simulink model "p5p5ex"  (Simulink 9.2)
settings: Solver=ode45  StartTime=0.0  StopTime=1000  RelTol=1e-3  EnableMultiTasking=on
values from neighbouring files (symbols this model uses):
  Kpd = 0.8427    [p5p5c.m]    (also in p5p5d.m; p5p5e.m)
  Td = T    (= 72.4391)    [p5p5c.m]    (also in p5p5d.m; p5p5e.m)
  Tf = 8.391    [p5p5c.m]    (also in p5p5d.m; p5p5e.m)
libraries: simulink x2
settings Model: Creator=markh  LastModifiedBy=Kevin K. Kaldvansvik
settings DataIOCC: SignalLoggingName=sigsOut
settings OptimizationCC: InitFltsAndDblsToZero=on
settings DebuggingCC: SaveWithParameterizedLinksMsg=none  SignalResolutionControl=TryResolveAllWithWarning  MultiTaskDSMMsg=warning  MultiTaskCondExecSysMsg=none
settings HardwareCC: TargetUnknown=on
settings GRTTargetCC: TargetFcnLib=ansi_tfl_tmw.mat

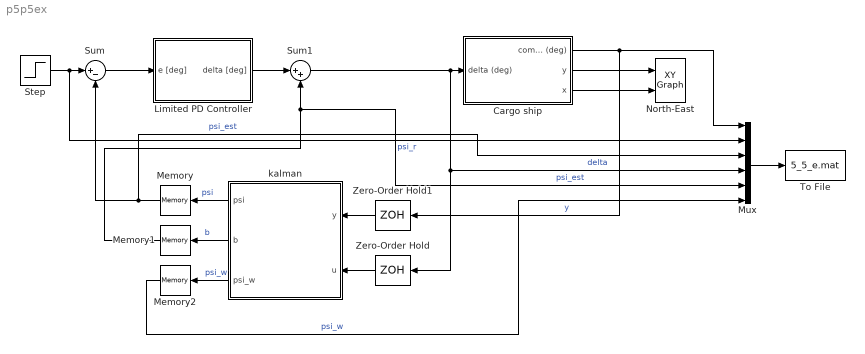
== system p5p5ex ==
  Cargo ship : Subsystem  mask(Simple shipmodel for a cargo ship){noise=on, current=on, logic=on}
      mask prompts: noise "measurement noise"; logic "waves"
      mask help:
      | Measurement noise:
      | 	checked = noise on
      | 	unchecked = noise off
      |
      | Current:
      | 	checked = current on
      | 	unchecked = current off
      |
      | Waves:
      | 	checked = waves on
      | 	unchecked = waves off
      |
      | Author: Jørgen Spjøtvold, 9/10-2003
      | TTK 4115 Linear system theory.
      | Modified by Jostein Bakkeheim 26/10-2006
  Limited PD Controller : Subsystem
  Memory : Memory
  Memory1 : Memory
  Memory2 : Memory
  Mux : Mux  Inputs=6
  North-East : simulink/Sinks/XY Graph  xmin=-5000  xmax=5000  ymin=-5000  ymax=5000  st=-1
  Step : Step  After=30  SampleTime=0
  Sum : Sum  Inputs=|+-
  Sum1 : Sum  Inputs=|++
  To File : ToFile  Filename=5_5_e.mat
  Zero-Order Hold : ZeroOrderHold  SampleTime=0.1
  Zero-Order Hold1 : ZeroOrderHold  SampleTime=0.1
  "kalman " : MATLAB Function  TreatAsAtomicUnit=on
  wires:
  Mux/1 -> To File/1
  Sum/1 -> Limited PD Controller/1(e [deg])
  Cargo ship/3(x) -> North-East/2
  Cargo ship/1(compass (deg)) -> Zero-Order Hold1/1, Mux/1  "y"
  Cargo ship/2(y) -> North-East/1
  "kalman "/1(psi) -> Memory/1  "psi"
  Zero-Order Hold/1 -> "kalman "/2(u)
  Zero-Order Hold1/1 -> "kalman "/1(y)
  "kalman "/2(b) -> Memory1/1  "b"
  Limited PD Controller/1(delta [deg]) -> Sum1/1
  Sum1/1 -> Zero-Order Hold/1, Mux/4, Cargo ship/1(delta (deg))  "delta"
  Step/1 -> Mux/2, Sum/1  "psi_r"
  Memory/1 -> Sum/2, Mux/3  "psi_est"
  Memory1/1 -> Mux/5, Sum1/2  "psi_est"
  "kalman "/3(psi_w) -> Memory2/1  "psi_w"
  Memory2/1 -> Mux/6  "psi_w"

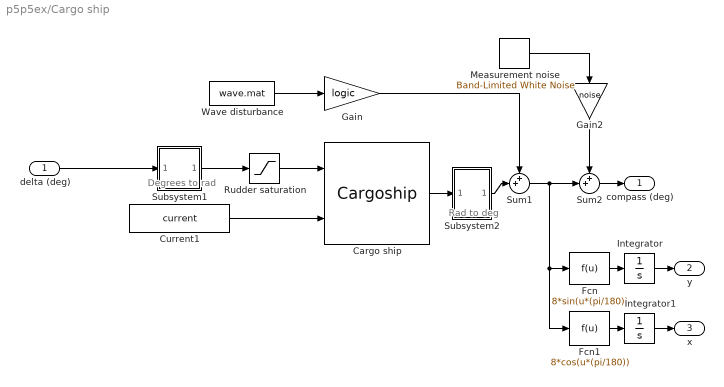
== system p5p5ex/Cargo ship ==
  note: Degrees to rad
  note: Rad to deg
  delta (deg) : Inport
  Cargo ship : S-Function  FunctionName=Cargoship  SFunctionDeploymentMode=off  EnableBusSupport=off  mask(Cargo ship){}
      mask help:
      | S-function which simulates a cargo ship.
      |
      | Author: Jørgen Spjøtvold
      | 20.10-2003
      | Modified by Jostein Bakkeheim 27.10.2006
  Current1 : Constant  Value=current
  Fcn : Fcn  Expr=8*sin(u*(pi/180))
  Fcn1 : Fcn  Expr=8*cos(u*(pi/180))
  Gain : Gain  Gain=logic  SaturateOnIntegerOverflow=on  OutDataTypeStr=Inherit: Same as input  ParamDataTypeStr=Inherit: Same as input
  Gain2 : Gain  Gain=noise  SaturateOnIntegerOverflow=on  OutDataTypeStr=Inherit: Same as input  ParamDataTypeStr=Inherit: Same as input
  Integrator : Integrator
  Integrator1 : Integrator
  Measurement noise : simulink/Sources/Band-Limited White Noise  Cov=[0.001]  Ts=.5  seed=[23341]
  Rudder saturation : Saturate  UpperLimit=45*(pi/180)  LowerLimit=-45*(pi/180)
  Subsystem1 : Subsystem  mask(degrees to radians){}
      mask help: Converts degrees to radians
      mask Display: fprintf('D2R');
  Subsystem2 : Subsystem  mask(radians to degrees){}
      mask help: Converts radians to degrees
      mask Display: fprintf('R2D');
  Sum1 : Sum  Inputs=++|  SaturateOnIntegerOverflow=on
  Sum2 : Sum  Inputs=++|  SaturateOnIntegerOverflow=on
  Wave disturbance : FromFile  FileName=wave.mat  SampleTime=0
  compass (deg) : Outport
  y : Outport  Port=2
  x : Outport  Port=3
  wires:
  delta (deg)/1 -> Subsystem1/1(In1)
  Fcn/1 -> Integrator/1
  Integrator/1 -> y/1
  Fcn1/1 -> Integrator1/1
  Integrator1/1 -> x/1
  Wave disturbance/1 -> Gain/1
  Subsystem2/1(Out1) -> Sum1/2
  Gain/1 -> Sum1/1
  Sum1/1 -> Fcn/1, Fcn1/1, Sum2/2
  Cargo ship/1 -> Subsystem2/1(In1)
  Subsystem1/1(Out1) -> Rudder saturation/1
  Rudder saturation/1 -> Cargo ship/1
  Sum2/1 -> compass (deg)/1
  Measurement noise/1 -> Gain2/1
  Gain2/1 -> Sum2/1
  Current1/1 -> Cargo ship/2

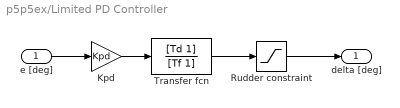
== system p5p5ex/Limited PD Controller ==
  e [deg] : Inport
  Kpd : Gain  Gain=Kpd
  Rudder constraint : Saturate  UpperLimit=45  LowerLimit=-45
  Transfer fcn : TransferFcn  Numerator=[Td 1]  Denominator=[Tf 1]
  delta [deg] : Outport
  wires:
  Kpd/1 -> Transfer fcn/1
  e [deg]/1 -> Kpd/1
  Transfer fcn/1 -> Rudder constraint/1
  Rudder constraint/1 -> delta [deg]/1

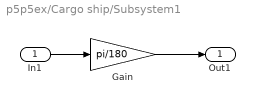
== system p5p5ex/Cargo ship/Subsystem1 ==
  In1 : Inport
  Gain : Gain  Gain=pi/180  SaturateOnIntegerOverflow=on  OutDataTypeStr=Inherit: Same as input  ParamDataTypeStr=Inherit: Same as input
  Out1 : Outport
  wires:
  Gain/1 -> Out1/1
  In1/1 -> Gain/1

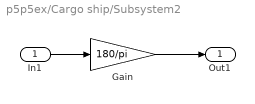
== system p5p5ex/Cargo ship/Subsystem2 ==
  In1 : Inport
  Gain : Gain  Gain=180/pi  SaturateOnIntegerOverflow=on  OutDataTypeStr=Inherit: Same as input  ParamDataTypeStr=Inherit: Same as input
  Out1 : Outport
  wires:
  Gain/1 -> Out1/1
  In1/1 -> Gain/1

== matlab function kalman  ==
  data: y input double; u input double; psi output double; b output double; psi_w output double
% Input: mÃ¥ling y, pÃ¥drag u
% Output: kalman filter: Estimert psi uten stÃ¸y og rudder bias b
function [psi, b, psi_w] = Kalman(y, u)

persistent  init_flag A B C E X_ R Q_k P_

% Initialize
if isempty(init_flag)
    
    init_flag = 1;
     
    Q_k = [1.68080996498622e-07,2.52832988209693e-06,0,0,0;
        2.52832988209693e-06,5.05671543189852e-05,0,0,0;
        0,0,2.32004646392527e-18,5.79922670073289e-17,-3.59028347101574e-13;
        0,0,5.79922670073289e-17,1.54628259912526e-15,-1.07696115999909e-11;
        0,0,-3.59028347101574e-13,-1.07696115999909e-11,1.00000000000000e-07];
    
    R = 0.00017326;

    P_0 =  [[1      0      0      0     0        ]
            [0      0.013  0      0     0        ]
            [0      0      pi^2   0     0        ]
            [0      0      0      1     0        ]
            [0      0      0      0     2.5*10^-3]];
        
    X_0 = [0 0 0 0 0]';
    
    A = [[0.996926739262672    0.100626789614164       0       0                    0                         ]
        [-0.061582920038110    1.011537233905485       0       0                    0                         ]
        [0                     0                       1       0.099931008253684    -1.076961159999087*10^-5  ]
        [0                     0                       0       0.998620482470742    -2.153426863171962*10^-4  ]
        [0                     0                       0       0                    1                         ]];
    
    B = [0 0 1.076961159999087*10^-5 2.153426863171962*10^-4 0]';
    
    C = [0 1 1 0 0];
    
    E = [[2.048850967535938*10^-5   4.105548994630666*10^-4     0                          0                            0                   ]
        [ 0                         0                           -3.590283471015735*10^-7   -1.076961159999087*10^-5     0.100000000000000   ]]';
    
    X_ = X_0;
    P_ = P_0;
end
%Kode som kjøres etter init av KF
    
%Omgjøring av input [deg] til [rad]
y = y.*(pi/180);
u = u.*(pi/180);

% [1] Computing the kalman gain L
L = P_*C.'*inv(C*P_*C.' + R);
    
% [2] Updating the estimate with the measurement y
X_hat = X_ + L * (y - C*X_);
    
% [3] Updating the error covariance matrix P
% This formula holds for both optimal and suboptimal gain L
P = (eye(5)- L*C) * P_ *(eye(5)-L*C).' + L*R*L.';
    
% [4] Projecting ahead
X_ = A*X_hat + B*u;
P_ = A*P*A.' + Q_k;

% Oppdaterer output heading psi og rudder bias b
% Konverterer også fra [rad] til [deg]
psi = X_hat(3).*(180/pi);
b = X_hat(5).*(180/pi);
psi_w = X_hat(2).*(180/pi);
end
